simulink model "test_brewery"  (R2023b)
settings: Solver=FixedStepAuto  StartTime=0  StopTime=18500  FixedStep=1  RelTol=1e-3
values from neighbouring files (symbols this model uses):
  A = 0.1817    [init_4_sim.m]    (also in startingThermodynamics.m)
  Cp = 1.2552    [init_4_sim.m]    (also in startingThermodynamics.m)
  delta_H = -91200    [init_4_sim.m]    (also in startingThermodynamics.m)
  h = 200.89    [init_4_sim.m]    (also in startingThermodynamics.m)
  rho = 1    [init_4_sim.m]    (also in startingThermodynamics.m)
  sug_current = sug_init    (= 1011.832)    [init_4_sim.m]    (also in init_sim2.m; init_sim_suggarferm.m)
  sug_init = 1011.832    [init_4_sim.m]    (also in init_sim.m = 1011; init_sim2.m; init_sim_suggarferm.m)
  t_cool = 293.15    [init_4_sim.m]
  T_k0 = 293.15    [init_4_sim.m]
  t_step = 1    [init_4_sim.m]    (also in init_sim2.m; init_sim_suggarferm.m; startingThermodynamics.m)
  temp = 296    [init_4_sim.m]    (also in init_sim.m = 298.15; init_sim2.m; init_sim_suggarferm.m)
  Vol = volume    (= 25)    [init_4_sim.m]    (also in startingThermodynamics.m)
  volume = 25    [init_4_sim.m]    (also in init_sim.m; init_sim2.m; init_sim_suggarferm.m)
  yeast_gram = 11    [init_4_sim.m]    (also in init_sim2.m; init_sim_suggarferm.m)
undefined symbols (not defined in the file or in its folder): A_amb, h_amb, T_amb
settings Model: Creator=20181234  LastModifiedBy=20181234

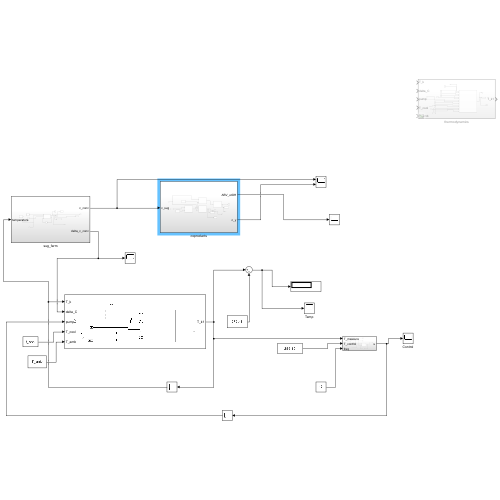
[thumbnail: Simulink's stored preview of the top-level diagram]
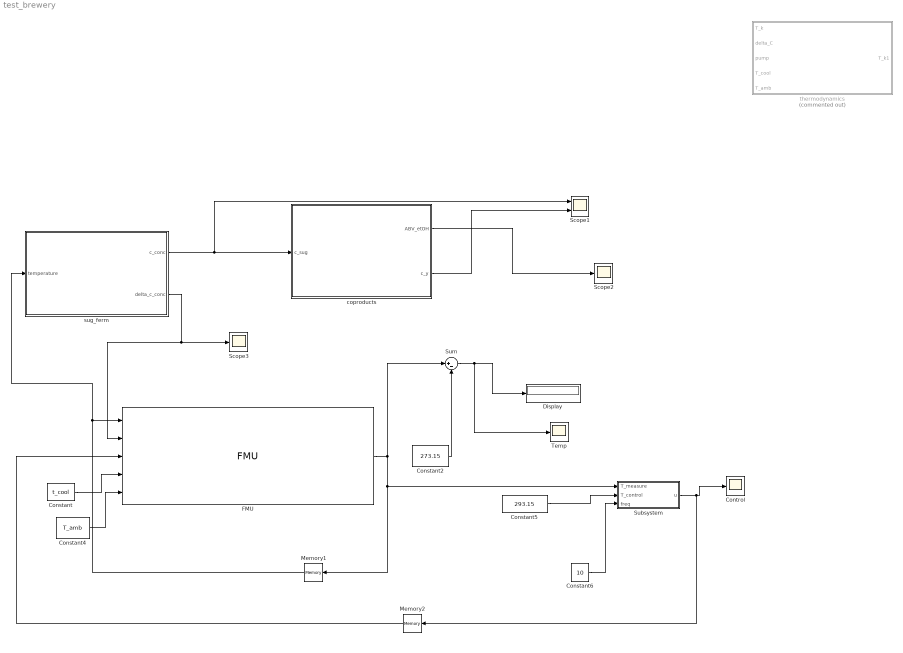
== system test_brewery ==
  Constant : Constant  Value=t_cool
  Constant2 : Constant  Value=273.15
  Constant4 : Constant  Value=T_amb
  Constant5 : Constant  Value=293.15
  Constant6 : Constant  Value=10
  Control : Scope
  Display : Display
  FMU : FMU  FMUName=ThermoDynamicsFMU.fmu  FMUMode=CoSimulation  FMUCreateBusObject=off  FMUInitializeEnumObject=off  FMUCachedDialogLayout="{\"Geometry\":[802,127,535,461],\"ParameterColumnsWidthConfig\":\"{\\\"columns\\\":[{\\\"name\\\":\\\"Parameter\\\",\\\"width\\\":140},{\\\"name\\\":\\\"Value\\\",\\\"width\\\":111},{\\\"name\\\":\\\"Unit\\\",\\\"width\\\":103},{\\\"name\\\":\\\"Description\\\",\\\"width\\\":144}]}\",\"InputColumnsWidthConfig\":[],\"OutputColumnsWidthConfig\":[]}"  A=0.31  A_amb=0.754  Cp=3.8  Vol=25  delta_H=-65  h=678.07  h_amb=42.93  rho=1000  t_step=1  mask(ThermoDynamicsFMU [Co-Simulation, v2.0]){}
      mask Display:
      | if (exist([Simulink.fileGenControl('get','CacheFolder') '\slprj\_fmu\08392b01092f6786554c1c071379a928\ThermoDynamicsFMU\model.png'],'file'))
      |     image([Simulink.fileGenControl('get','CacheFolder') '\slprj\_fmu\08392b01092f6786554c1c071379a928\ThermoDynamicsFMU\model.png']);
      | else
      |     disp('ThermoDynamicsFMU');
      | end
      | port_label('output',1,'T_k1');
      | port_label('input',1,'T_k');
      | port_label('input',2,'delta_C');
      | port_label('input',3,'pump');
      | port_label('input',4,'T_cool');
      | port_label('input',5,'T_amb');
  Memory1 : Memory  InitialCondition=T_k0
  Memory2 : Memory
  Scope1 : Scope  NumInputPorts=2
  Scope2 : Scope
  Scope3 : Scope
  Subsystem : Subsystem
  Sum : Sum  Inputs=|+-
  Temp : Scope
  coproducts : Subsystem
  sug_ferm : Subsystem
  thermodynamics : Subsystem  Commented=on
  wires:
  sug_ferm/1(c_conc) -> Scope1/1, coproducts/1(c_sug)
  sug_ferm/2(delta_c_conc) -> FMU/2, Scope3/1
  coproducts/1(ABV_etOH) -> Scope2/1
  coproducts/2(c_y) -> Scope1/2
  FMU/1 -> Sum/1, Memory1/1, Subsystem/1(T_measure)
  Memory1/1 -> sug_ferm/1(temperature), FMU/1
  Sum/1 -> Temp/1, Display/1
  Constant2/1 -> Sum/2
  Constant/1 -> FMU/4
  Constant4/1 -> FMU/5
  Constant5/1 -> Subsystem/2(T_control)
  Subsystem/1(u) -> Memory2/1, Control/1
  Memory2/1 -> FMU/3
  Constant6/1 -> Subsystem/3(freq)

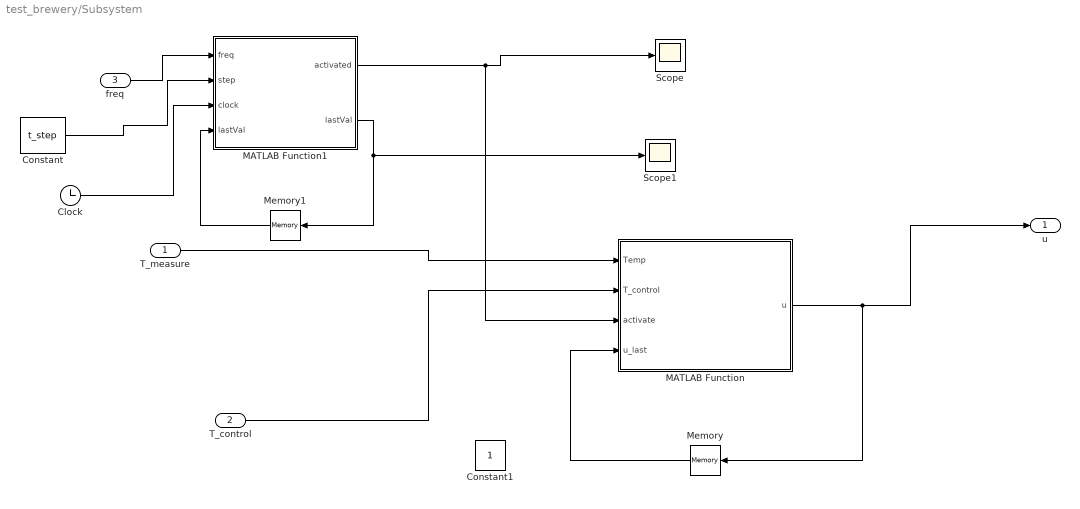
== system test_brewery/Subsystem ==
  T_measure : Inport
  T_control : Inport  Port=2
  freq : Inport  Port=3
  Clock : Clock
  Constant : Constant  Value=t_step
  Constant1 : Constant
  MATLAB Function : MATLAB Function  TreatAsAtomicUnit=on
  MATLAB Function1 : MATLAB Function  TreatAsAtomicUnit=on
  Memory : Memory  LinearizeAsDelay=on
  Memory1 : Memory
  Scope : Scope
  Scope1 : Scope
  u : Outport
  wires:
  T_control/1 -> MATLAB Function/2(T_control)
  T_measure/1 -> MATLAB Function/1(Temp)
  MATLAB Function/1(u) -> Memory/1, u/1
  Clock/1 -> MATLAB Function1/3(clock)
  MATLAB Function1/1(activated) -> MATLAB Function/3(activate), Scope/1
  Memory/1 -> MATLAB Function/4(u_last)
  Constant/1 -> MATLAB Function1/2(step)
  freq/1 -> MATLAB Function1/1(freq)
  MATLAB Function1/2(lastVal) -> Memory1/1, Scope1/1
  Memory1/1 -> MATLAB Function1/4("lastVal ")

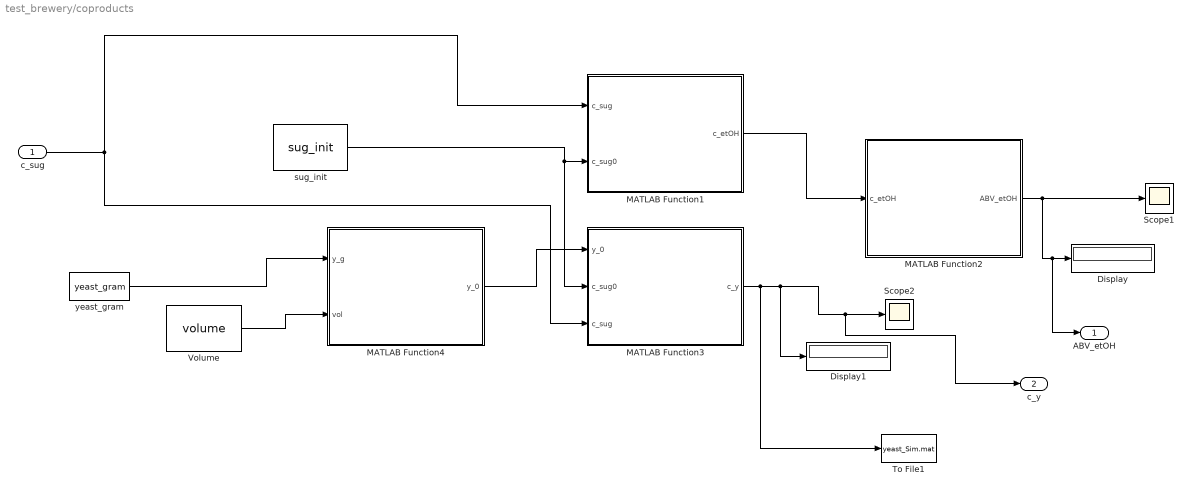
== system test_brewery/coproducts ==
  c_sug : Inport
  Display : Display
  Display1 : Display
  MATLAB Function1 : MATLAB Function  TreatAsAtomicUnit=on
  MATLAB Function2 : MATLAB Function  TreatAsAtomicUnit=on
  MATLAB Function3 : MATLAB Function  TreatAsAtomicUnit=on
  MATLAB Function4 : MATLAB Function  TreatAsAtomicUnit=on
  Scope1 : Scope
  Scope2 : Scope
  To File1 : ToFile  Filename=yeast_Sim.mat  MatrixName=yeast
      settings: Decimation=2
  Volume : Constant  Value=volume
  sug_init : Constant  Value=sug_init
  yeast_gram : Constant  Value=yeast_gram
  ABV_etOH : Outport
  c_y : Outport  Port=2
  wires:
  yeast_gram/1 -> MATLAB Function4/1(y_g)
  MATLAB Function3/1(c_y) -> To File1/1, Display1/1, c_y/1, Scope2/1
  c_sug/1 -> MATLAB Function3/3(c_sug), MATLAB Function1/1(c_sug)
  MATLAB Function1/1(c_etOH) -> MATLAB Function2/1(c_etOH)
  MATLAB Function2/1(ABV_etOH) -> ABV_etOH/1, Display/1, Scope1/1
  MATLAB Function4/1(y_0) -> MATLAB Function3/1(y_0)
  sug_init/1 -> MATLAB Function3/2(c_sug0), MATLAB Function1/2(c_sug0)
  Volume/1 -> MATLAB Function4/2(vol)

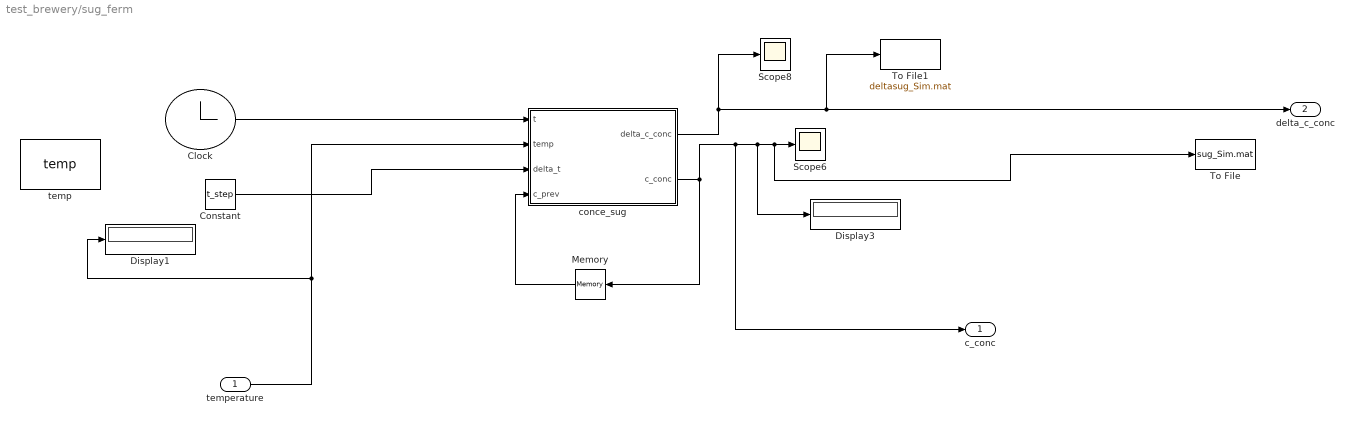
== system test_brewery/sug_ferm ==
  temperature : Inport
  Clock : Clock
  Constant : Constant  Value=t_step
  Display1 : Display
  Display3 : Display
  Memory : Memory  InitialCondition=sug_current
  Scope6 : Scope
  Scope8 : Scope
  To File : ToFile  Filename=sug_Sim.mat  MatrixName=sug_conc
  To File1 : ToFile  Filename=deltasug_Sim.mat  MatrixName=sug_conc
  conce_sug : Subsystem
  temp : Constant  Value=temp
  c_conc : Outport
  delta_c_conc : Outport  Port=2
  wires:
  Memory/1 -> conce_sug/4(c_prev)
  conce_sug/1(delta_c_conc) -> Scope8/1, To File1/1, delta_c_conc/1
  Clock/1 -> conce_sug/1(t)
  conce_sug/2(c_conc) -> Memory/1, c_conc/1, Display3/1, To File/1, Scope6/1
  Constant/1 -> conce_sug/3(delta_t)
  temperature/1 -> Display1/1, conce_sug/2(temp)

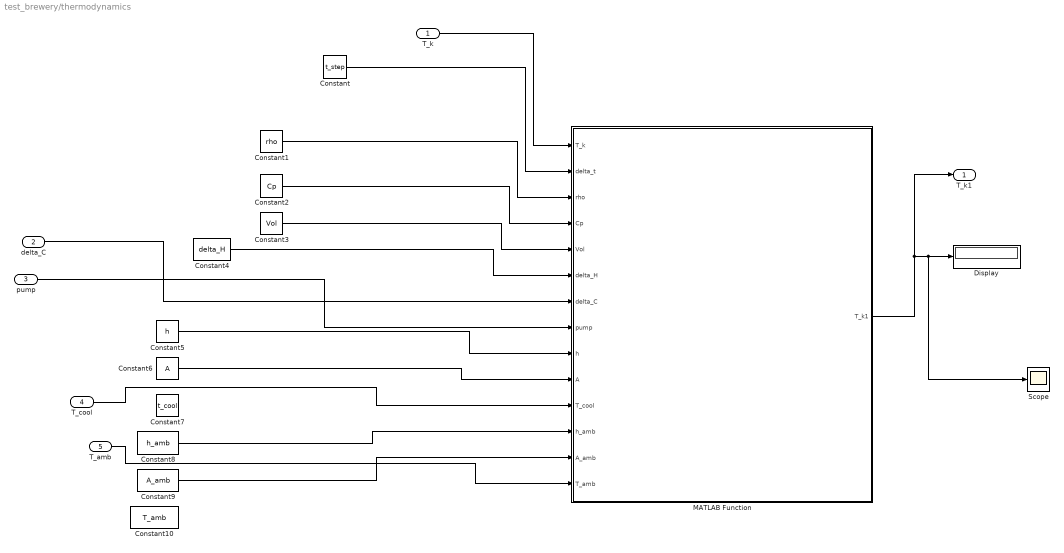
== system test_brewery/thermodynamics ==
  T_k : Inport
  delta_C : Inport  Port=2
  pump : Inport  Port=3
  T_cool : Inport  Port=4
  T_amb : Inport  Port=5
  Constant : Constant  Value=t_step
  Constant1 : Constant  Value=rho
  Constant10 : Constant  Value=T_amb
  Constant2 : Constant  Value=Cp
  Constant3 : Constant  Value=Vol
  Constant4 : Constant  Value=delta_H
  Constant5 : Constant  Value=h
  Constant6 : Constant  Value=A
  Constant7 : Constant  Value=t_cool
  Constant8 : Constant  Value=h_amb
  Constant9 : Constant  Value=A_amb
  Display : Display
  MATLAB Function : MATLAB Function  TreatAsAtomicUnit=on
  Scope : Scope
  T_k1 : Outport
  wires:
  Constant4/1 -> MATLAB Function/6(delta_H)
  delta_C/1 -> MATLAB Function/7(delta_C)
  Constant5/1 -> MATLAB Function/9(h)
  Constant6/1 -> MATLAB Function/10(A)
  Constant1/1 -> MATLAB Function/3(rho)
  MATLAB Function/1(T_k1) -> T_k1/1, Scope/1, Display/1
  pump/1 -> MATLAB Function/8(pump)
  Constant2/1 -> MATLAB Function/4(Cp)
  Constant3/1 -> MATLAB Function/5(Vol)
  Constant/1 -> MATLAB Function/2(delta_t)
  T_k/1 -> MATLAB Function/1(T_k)
  Constant8/1 -> MATLAB Function/12(h_amb)
  Constant9/1 -> MATLAB Function/13(A_amb)
  T_cool/1 -> MATLAB Function/11(T_cool)
  T_amb/1 -> MATLAB Function/14(T_amb)

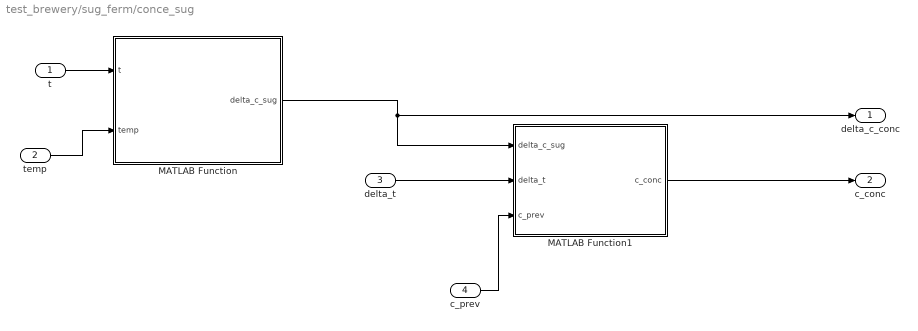
== system test_brewery/sug_ferm/conce_sug ==
  t : Inport
  temp : Inport  Port=2
  delta_t : Inport  Port=3
  c_prev : Inport  Port=4
  MATLAB Function : MATLAB Function  TreatAsAtomicUnit=on
  MATLAB Function1 : MATLAB Function  TreatAsAtomicUnit=on
  delta_c_conc : Outport
  c_conc : Outport  Port=2
  wires:
  MATLAB Function/1(delta_c_sug) -> delta_c_conc/1, MATLAB Function1/1(delta_c_sug)
  MATLAB Function1/1(c_conc) -> c_conc/1
  t/1 -> MATLAB Function/1(t)
  temp/1 -> MATLAB Function/2(temp)
  delta_t/1 -> MATLAB Function1/2(delta_t)
  c_prev/1 -> MATLAB Function1/3(c_prev)

== matlab function test_brewery/coproducts/MATLAB Function1 ==
  data: c_sug input; c_etOH output; c_sug0 input
function c_etOH = conc_etOH(c_sug,c_sug0)
%stequimetry
st= 1.503;
%st= 1.5075;



c_etOH = (c_sug0-c_sug)*st;

== matlab function test_brewery/thermodynamics/MATLAB Function ==
  data: T_k input; T_k1 output; delta_t input; rho input; Cp input; Vol input; delta_H input; delta_C input; pump input; h input; A input; T_cool input; h_amb input; A_amb input; T_amb input
function T_k1 = thermo(T_k,delta_t, rho, Cp, Vol, delta_H, delta_C, pump, h, A, T_cool,h_amb, A_amb, T_amb)


factor = delta_t / (rho * Cp * (Vol/1000));
T_k1 = factor * (delta_H * delta_C*Vol - pump * h *60/1000 * A * (T_k - T_cool)-h_amb *60/1000 * A_amb * (T_k - T_amb)) + T_k;

== matlab function test_brewery/coproducts/MATLAB Function2 ==
  data: c_etOH input; ABV_etOH output
function ABV_etOH = ABV(c_etOH)
%stequimetry
MW_etOH = 46;%mol/g
density_etOH = 0.789; %g/ml




ABV_etOH = c_etOH*(MW_etOH/density_etOH)/1000^2*100;

== matlab function test_brewery/coproducts/MATLAB Function3 ==
  data: y_0 input; c_sug0 input; c_sug input; c_y output
function c_y = conc_yeast(y_0,c_sug0,c_sug)
%stequimetry
Y_trans = 0.1;
MW_sug = 180.16; %g/mol
MW_y = 24; %g/mol



c_y = (c_sug0-c_sug)*(MW_sug/MW_y)*Y_trans+y_0;

== matlab function test_brewery/coproducts/MATLAB Function4 ==
  data: y_g input; vol input; y_0 output
function y_0 = y_init(y_g,vol)

MW_y = 24; %g/mol


y_0 = (y_g/(vol*1000))/MW_y;

== matlab function test_brewery/sug_ferm/conce_sug/MATLAB Function ==
  data: t input; delta_c_sug output; temp input
function delta_c_sug = dela_conc_sug(t,temp)
A = 1.24503386e-22;
E = -9.35902242e4;
m = -0.000132816;
b = -0.058764065;
R = 8.314; %j/molK

c1=A*exp(-E/(R*temp));
c2=m*temp + b;

delta_c_sug = 2*c1*t+c2;
if delta_c_sug >= 0
    delta_c_sug = 0;
end

== matlab function test_brewery/sug_ferm/conce_sug/MATLAB Function1 ==
  data: delta_c_sug input; c_conc output; delta_t input; c_prev input
function c_conc = c_conc_func(delta_c_sug, delta_t,c_prev)

c_conc = c_prev + delta_t*delta_c_sug;

== matlab function test_brewery/Subsystem/MATLAB Function ==
  data: Temp input; u output; T_control input; activate input; u_last input
function u = controlLogic(Temp, T_control, activate, u_last)

if activate == true

    if Temp>= T_control
        u = 1;
    else
        u=0;
    end
else
    u= u_last;
end

== matlab function test_brewery/Subsystem/MATLAB Function1 ==
  data: freq input; activated output; step input; clock input; lastVal output; lastVal input
function [activated, lastVal]= activate_control(freq, step, clock, lastVal)



if clock == 0 || lastVal <= 0
    activated  = true;
    lastVal = freq;
else
    %lastVal = lastVal-step;
    activated = false;
end

lastVal = lastVal-step;
